simulink model "Control_Phase_Model"  (R2025b)
settings: Solver=ode4  StartTime=0.0  StopTime=10  FixedStep=0.001  RelTol=1e-3
undefined symbols (not defined in the file): b, j, km, l, mu, r
settings Model: Creator=moata  LastModifiedBy=moata

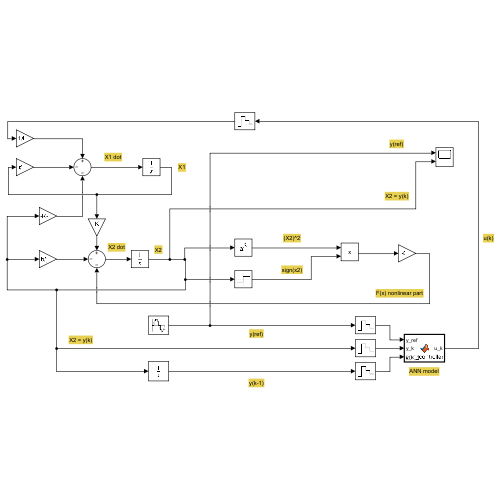
[thumbnail: Simulink's stored preview of the top-level diagram]
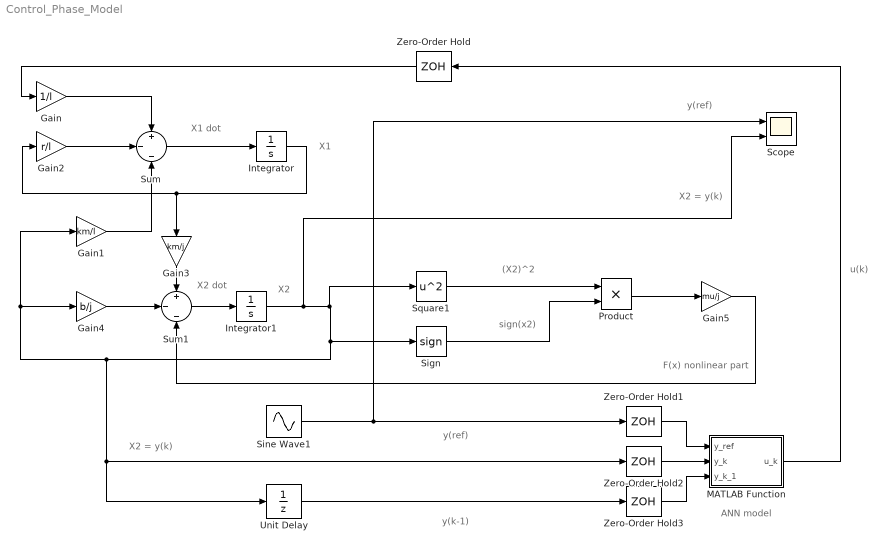
== system Control_Phase_Model ==
  note: X1
  note: X1 dot
  note: X2 dot
  note: X2
  note: (X2)^2
  note: sign(x2)
  note: F(x) nonlinear part
  note: u(k)
  note: X2 = y(k)
  note: y(k-1)
  note: y(ref)
  note: ANN model
  note: y(ref)
  note: X2 = y(k)
  Gain : Gain  Gain=1/l
  Gain1 : Gain  Gain=km/l
  Gain2 : Gain  Gain=r/l
  Gain3 : Gain  Gain=km/j
  Gain4 : Gain  Gain=b/j
  Gain5 : Gain  Gain=mu/j
  Integrator : Integrator
  Integrator1 : Integrator
  MATLAB Function : MATLAB Function  TreatAsAtomicUnit=on
  Product : Product
  Scope : Scope  NumInputPorts=2
      settings: ActiveDisplayYMinimum=-12.49363804589699  ActiveDisplayYMaximum=12.493119894584058
  Sign : Signum
  Sine Wave1 : Sin  Amplitude=10  Frequency=3.14  SampleTime=0.04
  Square1 : Math  Operator=square
  Sum : Sum  Inputs=+|-|-
  Sum1 : Sum  Inputs=+|-|-
  Unit Delay : UnitDelay  SampleTime=0.04  HasFrameUpgradeWarning=on
  Zero-Order Hold{,1..3} (4 alike) : ZeroOrderHold  SampleTime=0.04
  wires:
  Sum/1 -> Integrator/1
  Square1/1 -> Product/1
  Product/1 -> Gain5/1
  Gain2/1 -> Sum/2
  Gain4/1 -> Sum1/2
  Integrator/1 -> Gain3/1, Gain2/1
  Unit Delay/1 -> Zero-Order Hold3/1
  Gain1/1 -> Sum/3
  Integrator1/1 -> Unit Delay/1, Zero-Order Hold2/1, Gain4/1, Gain1/1, Sign/1, Square1/1, Scope/2
  Sign/1 -> Product/2
  Gain/1 -> Sum/1
  Sum1/1 -> Integrator1/1
  Gain3/1 -> Sum1/1
  MATLAB Function/1(u_k) -> Zero-Order Hold/1
  Zero-Order Hold/1 -> Gain/1
  Gain5/1 -> Sum1/3
  Sine Wave1/1 -> Zero-Order Hold1/1, Scope/1
  Zero-Order Hold1/1 -> MATLAB Function/1(y_ref)
  Zero-Order Hold2/1 -> MATLAB Function/2(y_k)
  Zero-Order Hold3/1 -> MATLAB Function/3(y_k_1)

== matlab function Control_Phase_Model/MATLAB Function ==
  data: y_ref input; u_k output; y_k input; y_k_1 input
function u_k = ann_controller(y_ref, y_k, y_k_1)
% This function implements the ANN Controller
% Based on the equation: u(k) = f(y_ref(k), y(k), y(k-1))

% Tell Simulink not to compile these Python functions
coder.extrinsic('py.importlib.import_module');
coder.extrinsic('py.joblib.load');
coder.extrinsic('py.numpy.array');
coder.extrinsic('py.numpy.reshape');
coder.extrinsic('py.tuple');
coder.extrinsic('int32'); % For creating the reshape tuple

% --- Initialize output to define its size and type ---
u_k = 0.0;

% Use persistent variables
persistent scaler model reshaper_tuple;

% Load the model on the first step
if isempty(model)
    py.importlib.import_module('joblib');
    py.importlib.import_module('numpy');
    
    scaler = py.joblib.load('ann_identifier_scaler.pkl');
    model = py.joblib.load('ann_identifier_model.pkl');
    
    % Create the constant reshape tuple (1, -1)
    reshaper_tuple = py.tuple([int32(1), int32(-1)]);
    
    disp('Python ANN model and scaler loaded into Simulink.');
end

% --- Step 1. Format Inputs ---
X_live = [y_ref, y_k, y_k_1];

% Convert to a 1D Python (Numpy) array
X_py_1d = py.numpy.array(X_live);

% Reshape to 2D numpy array [1, 3]
X_py = py.numpy.reshape(X_py_1d, reshaper_tuple);

% --- Step 2. Scale the Inputs ---
% This will now work, as the scaler expects a NumPy array
X_scaled = feval('transform', scaler, X_py);

% --- Step 3. Predict the Control Signal ---
u_k_py = feval('predict', model, X_scaled);

% --- Step 4. Return the Output ---
u_k = double(u_k_py);

end
